simulink model "sampleModel1564"  (R2023a)
settings: Solver=VariableStepAuto  StartTime=0.0  StopTime=10.0  RelTol=1e-3
libraries: hdlsllib x7, simulink x3
settings Model: Creator=user1  LastModifiedBy=user1

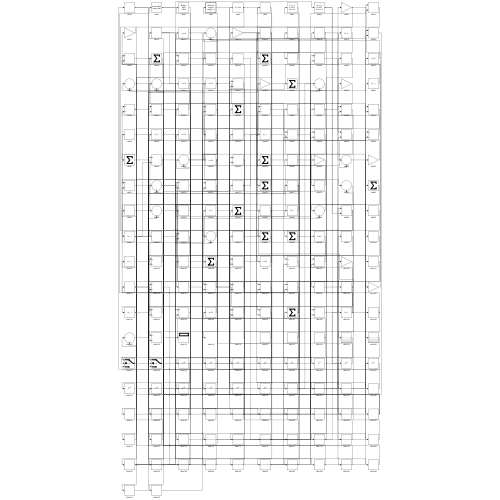
[thumbnail: Simulink's stored preview of the top-level diagram]
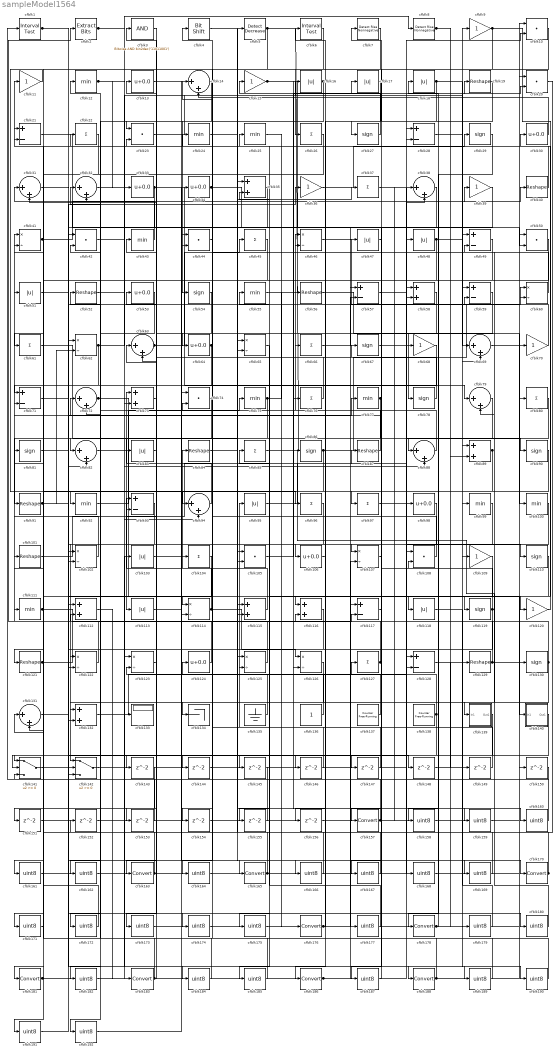
== system sampleModel1564 ==
  cfblk1 : hdlsllib/Logic and Bit Operations/Interval Test  IntervalClosedRight=on  uplimit=0.5  IntervalClosedLeft=on  lowlimit=-0.5  OutDataTypeStr=boolean
  cfblk{10,20,23,42,44,50,74,105,108} (9 alike) : DotProduct  OutDataTypeStr=Inherit: Inherit via internal rule
  cfblk{12,24..25,43,55,75,77,92,99..100,111} (11 alike) : MinMax
  cfblk{19,40,52,56,84,87,91,101,121,129} (10 alike) : Reshape
  cfblk{41,46,60,62,65,102,107,114,122..123,125..126} (12 alike) : Product  Inputs=*/  RndMeth=Zero  SaturateOnIntegerOverflow=on
  cfblk{16..18,47..48,51,83,95,103,113,118} (11 alike) : Abs  SaturateOnIntegerOverflow=off
  cfblk{22,26,37,45,61,66,76,80,85,96..97,104,127} (13 alike) : Sum  Inputs=+
  cfblk{13,30,33..34,53,64,98,106,124} (9 alike) : Bias  Bias=0.0  SaturateOnIntegerOverflow=off
  cfblk{9,11,15,36,39,68,70,109,120} (9 alike) : Gain
  cfblk{27,29,54,67,78,81,86,90,110,119,130} (11 alike) : Signum
  cfblk{35,58,73,89,112,115..116,132} (8 alike) : Sum
  cfblk{21,28,49,57,59,71,93,117,128} (9 alike) : Sum  Inputs=+-
  cfblk{14,31..32,38,63,69,72,79,82,88,94,131} (12 alike) : Sum  Inputs=|++
  cfblk133 : Display
  cfblk134 : Terminator
  cfblk135 : Ground
  cfblk136 : Constant  SampleTime=-1
  cfblk137 : hdlsllib/Sources/Counter Free-Running  NumBits=16  tsamp=-1
  cfblk138 : hdlsllib/Sources/Counter Free-Running  NumBits=16  tsamp=-1
  cfblk139 : Subsystem
      settings: LibrarySourceBlock=|
      | hdlsllib/Ports &
      | Subsystems/Subsystem
  cfblk140 : Subsystem
      settings: LibrarySourceBlock=|
      | hdlsllib/Ports &
      | Subsystems/Subsystem
  cfblk141 : Switch  SaturateOnIntegerOverflow=off  InputSameDT=off
  cfblk142 : Switch  SaturateOnIntegerOverflow=off  InputSameDT=off
  cfblk{143..156} (14 alike) : Delay  SampleTime=1
  cfblk{157,163,165,170,176,178,181,183,186,188} (10 alike) : DataTypeConversion  SaturateOnIntegerOverflow=off  RndMeth=Floor
  cfblk{158..162,164,166..169,171..175,177,179..180,182,184..185,187,189..192} (26 alike) : DataTypeConversion  OutDataTypeStr=uint8  SaturateOnIntegerOverflow=off  RndMeth=Floor
  cfblk2 : simulink/Logic and Bit Operations/Extract Bits  bitsToExtract=Upper half  numBits=8  bitIdxRange=[0 7]  outScalingMode=Preserve fixed-point scaling
      settings: LibrarySourceBlock=|
      | hdlsllib/Logic and Bit
      | Operations/Extract Bits
  cfblk3 : simulink/Logic and Bit Operations/Bitwise Operator  logicop=AND  UseBitMask=on  BitMask=bin2dec('11011001')  BitMaskRealWorld=Stored Integer
      settings: LibrarySourceBlock=|
      | hdlsllib/Logic and Bit
      | Operations/Bitwise
      | Operator
  cfblk4 : hdlsllib/Logic and Bit Operations/Bit Shift  mode=Shift Left Logical  N=0
  cfblk5 : simulink/Logic and Bit Operations/Detect Decrease  vinit=0.0  OutDataTypeStr=boolean
      settings: LibrarySourceBlock=|
      | hdlsllib/Logic and Bit
      | Operations/Detect
      | Decrease
  cfblk6 : hdlsllib/Logic and Bit Operations/Interval Test  IntervalClosedRight=on  uplimit=0.5  IntervalClosedLeft=on  lowlimit=-0.5  OutDataTypeStr=boolean
  cfblk7 : hdlsllib/Logic and Bit Operations/Detect Rise Nonnegative  vinit=0  OutDataTypeStr=boolean
  cfblk8 : hdlsllib/Logic and Bit Operations/Detect Rise Nonnegative  vinit=0  OutDataTypeStr=boolean
  wires:
  cfblk82/1 -> cfblk119/1
  cfblk47/1 -> cfblk97/1
  cfblk41/1 -> cfblk40/1, cfblk21/2
  cfblk40/1 -> cfblk11/1
  cfblk11/1 -> cfblk92/1
  cfblk125/1 -> cfblk2/1
  cfblk135/1 -> cfblk95/1
  cfblk122/1 -> cfblk41/1
  cfblk109/1 -> cfblk157/1
  cfblk63/1 -> cfblk45/1, cfblk59/2
  cfblk121/1 -> cfblk21/1, cfblk65/2, cfblk81/1
  cfblk85/1 -> cfblk139/1(In1)
  cfblk36/1 -> cfblk29/1
  cfblk32/1 -> cfblk188/1
  cfblk86/1 -> cfblk60/1, cfblk154/1
  cfblk96/1 -> cfblk142/1
  cfblk55/1 -> cfblk39/1
  cfblk37/1 -> cfblk110/1
  cfblk114/1 -> cfblk126/1, cfblk93/1, cfblk37/1
  cfblk77/1 -> cfblk113/1, cfblk71/2
  cfblk124/1 -> cfblk43/1
  cfblk12/1 -> cfblk33/1, cfblk88/2, cfblk174/1
  cfblk5/1 -> cfblk86/1, cfblk63/2
  cfblk115/1 -> cfblk84/1
  cfblk44/1 -> cfblk134/1
  cfblk26/1 -> cfblk121/1
  cfblk9/1 -> cfblk120/1, cfblk27/1
  cfblk126/1 -> cfblk132/1
  cfblk19/1 -> cfblk106/1
  cfblk102/1 -> cfblk51/1
  cfblk88/1 -> cfblk46/1
  cfblk78/1 -> cfblk46/2
  cfblk87/1 -> cfblk12/1
  cfblk91/1 -> cfblk62/1, cfblk62/2, cfblk96/1
  cfblk129/1 -> cfblk10/1, cfblk108/2, cfblk55/1
  cfblk120/1 -> cfblk30/1
  cfblk70/1 -> cfblk47/1
  cfblk105/1 -> cfblk19/1
  cfblk25/1 -> cfblk176/1
  cfblk95/1 -> cfblk87/1
  cfblk52/1 -> cfblk123/1
  cfblk29/1 -> cfblk88/1
  cfblk45/1 -> cfblk82/1
  cfblk17/1 -> cfblk186/1
  cfblk69/1 -> cfblk100/1
  cfblk119/1 -> cfblk7/1, cfblk79/2, cfblk142/3, cfblk155/1
  cfblk28/1 -> cfblk69/1
  cfblk123/1 -> cfblk53/1
  cfblk49/1 -> cfblk178/1
  cfblk16/1 -> cfblk126/2, cfblk122/1
  cfblk83/1 -> cfblk13/1
  cfblk97/1 -> cfblk128/1
  cfblk48/1 -> cfblk61/1, cfblk20/2
  cfblk61/1 -> cfblk125/1
  cfblk21/1 -> cfblk76/1
  cfblk43/1 -> cfblk31/1
  cfblk33/1 -> cfblk79/1, cfblk132/2
  cfblk76/1 -> cfblk31/2
  cfblk111/1 -> cfblk117/2, cfblk77/1
  cfblk2/1 -> cfblk8/1, cfblk189/1
  cfblk15/1 -> cfblk57/1, cfblk160/1
  cfblk8/1 -> cfblk89/2, cfblk149/1
  cfblk72/1 -> cfblk140/1(In1), cfblk94/2
  cfblk112/1 -> cfblk183/1
  cfblk59/1 -> cfblk78/1
  cfblk7/1 -> cfblk26/1
  cfblk90/1 -> cfblk128/2
  cfblk34/1 -> cfblk59/1, cfblk164/1
  cfblk60/1 -> cfblk4/1
  cfblk94/1 -> cfblk73/1
  cfblk132/1 -> cfblk28/1
  cfblk81/1 -> cfblk60/2
  cfblk1/1 -> cfblk116/1, cfblk180/1
  cfblk3/1 -> cfblk23/1
  cfblk18/1 -> cfblk50/2, cfblk156/1
  cfblk80/1 -> cfblk118/1
  cfblk56/1 -> cfblk80/1
  cfblk62/1 -> cfblk16/1, cfblk71/1
  cfblk14/1 -> cfblk54/1
  cfblk136/1 -> cfblk123/2
  cfblk92/1 -> cfblk34/1
  cfblk130/1 -> cfblk35/2, cfblk185/1
  cfblk89/1 -> cfblk141/1, cfblk105/2
  cfblk64/1 -> cfblk122/2, cfblk162/1
  cfblk38/1 -> cfblk73/2
  cfblk39/1 -> cfblk107/1
  cfblk27/1 -> cfblk15/1
  cfblk137/1 -> cfblk127/1
  cfblk141/1 -> cfblk36/1
  cfblk101/1 -> cfblk10/2
  cfblk84/1 -> cfblk5/1
  cfblk106/1 -> cfblk6/1
  cfblk23/1 -> cfblk9/1
  cfblk35/1 -> cfblk83/1
  cfblk10/1 -> cfblk64/1
  cfblk68/1 -> cfblk181/1
  cfblk57/1 -> cfblk90/1
  cfblk128/1 -> cfblk69/2
  cfblk138/1 -> cfblk23/2, cfblk141/2
  cfblk50/1 -> cfblk114/1
  cfblk74/1 -> cfblk91/1
  cfblk131/1 -> cfblk170/1
  cfblk99/1 -> cfblk163/1
  cfblk127/1 -> cfblk41/2, cfblk85/1
  cfblk142/1 -> cfblk65/1
  cfblk93/1 -> cfblk142/2
  cfblk71/1 -> cfblk94/1
  cfblk103/1 -> cfblk75/1
  cfblk54/1 -> cfblk114/2
  cfblk108/1 -> cfblk74/2
  cfblk30/1 -> cfblk14/2
  cfblk42/1 -> cfblk165/1
  cfblk66/1 -> cfblk57/2
  cfblk75/1 -> cfblk102/2, cfblk56/1
  cfblk73/1 -> cfblk143/1
  cfblk51/1 -> cfblk144/1
  cfblk144/1 -> cfblk28/2
  cfblk65/1 -> cfblk145/1
  cfblk145/1 -> cfblk1/1
  cfblk98/1 -> cfblk146/1
  cfblk146/1 -> cfblk125/2
  cfblk107/1 -> cfblk147/1
  cfblk147/1 -> cfblk117/1
  cfblk13/1 -> cfblk148/1
  cfblk149/1 -> cfblk14/1
  cfblk150/1 -> cfblk141/3
  cfblk6/1 -> cfblk151/1
  cfblk151/1 -> cfblk89/1
  cfblk20/1 -> cfblk152/1
  cfblk152/1 -> cfblk74/1
  cfblk140/1(Out1) -> cfblk153/1
  cfblk153/1 -> cfblk72/1
  cfblk154/1 -> cfblk115/2
  cfblk155/1 -> cfblk63/1
  cfblk156/1 -> cfblk116/2
  cfblk157/1 -> cfblk20/1, cfblk105/1, cfblk38/1
  cfblk139/1(Out1) -> cfblk158/1
  cfblk158/1 -> cfblk109/1
  cfblk24/1 -> cfblk159/1
  cfblk159/1 -> cfblk50/1
  cfblk160/1 -> cfblk24/1
  cfblk22/1 -> cfblk161/1
  cfblk161/1 -> cfblk108/1
  cfblk162/1 -> cfblk22/1
  cfblk163/1 -> cfblk72/2, cfblk3/1
  cfblk164/1 -> cfblk99/1
  cfblk165/1 -> cfblk35/1, cfblk101/1, cfblk38/2
  cfblk4/1 -> cfblk166/1
  cfblk166/1 -> cfblk42/1
  cfblk79/1 -> cfblk167/1
  cfblk167/1 -> cfblk42/2
  cfblk67/1 -> cfblk168/1
  cfblk168/1 -> cfblk70/1
  cfblk113/1 -> cfblk169/1
  cfblk169/1 -> cfblk67/1
  cfblk170/1 -> cfblk52/1, cfblk44/1, cfblk115/1
  cfblk143/1 -> cfblk171/1
  cfblk171/1 -> cfblk131/1
  cfblk116/1 -> cfblk172/1
  cfblk172/1 -> cfblk131/2
  cfblk58/1 -> cfblk173/1
  cfblk173/1 -> cfblk48/1
  cfblk174/1 -> cfblk58/1
  cfblk110/1 -> cfblk175/1
  cfblk175/1 -> cfblk58/2
  cfblk176/1 -> cfblk150/1, cfblk66/1
  cfblk46/1 -> cfblk177/1
  cfblk177/1 -> cfblk25/1
  cfblk178/1 -> cfblk18/1, cfblk129/1
  cfblk118/1 -> cfblk179/1
  cfblk179/1 -> cfblk49/1
  cfblk180/1 -> cfblk49/2
  cfblk181/1 -> cfblk133/1, cfblk103/1, cfblk44/2, cfblk82/2
  cfblk53/1 -> cfblk182/1
  cfblk182/1 -> cfblk68/1
  cfblk183/1 -> cfblk93/2, cfblk111/1
  cfblk31/1 -> cfblk184/1
  cfblk184/1 -> cfblk112/1
  cfblk185/1 -> cfblk112/2
  cfblk186/1 -> cfblk107/2, cfblk98/1
  cfblk117/1 -> cfblk187/1
  cfblk187/1 -> cfblk17/1
  cfblk188/1 -> cfblk124/1, cfblk130/1
  cfblk189/1 -> cfblk32/1
  cfblk148/1 -> cfblk190/1
  cfblk190/1 -> cfblk32/2
  cfblk104/1 -> cfblk191/1
  cfblk191/1 -> cfblk102/1
  cfblk100/1 -> cfblk192/1
  cfblk192/1 -> cfblk104/1

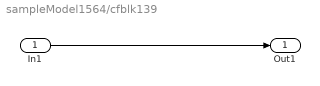
== system sampleModel1564/cfblk139 ==
  In1 : Inport
  Out1 : Outport
  wires:
  In1/1 -> Out1/1

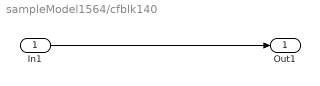
== system sampleModel1564/cfblk140 ==
  In1 : Inport
  Out1 : Outport
  wires:
  In1/1 -> Out1/1
